simulink model "Sim_model"  (R2022b)
settings: Solver=daessc  StartTime=0.0  StopTime=10.0  RelTol=1e-5
settings Model: Creator=theko  LastModifiedBy=theko

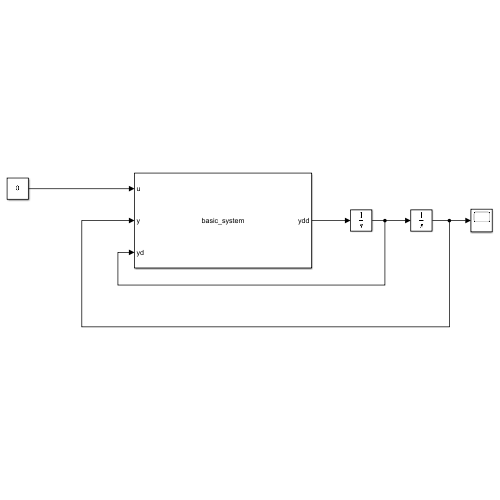
[thumbnail: Simulink's stored preview of the top-level diagram]
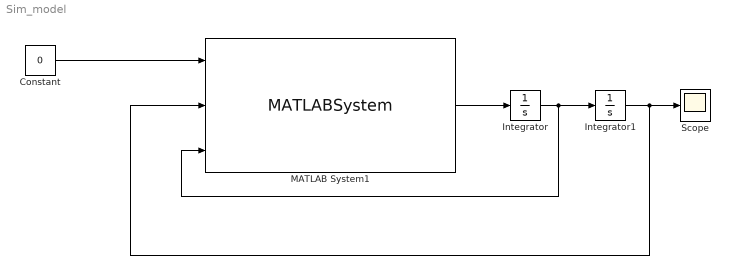
== system Sim_model ==
  Constant : Constant  Value=0
  Integrator : Integrator  InitialCondition=1
  Integrator1 : Integrator  InitialCondition=1
  MATLAB System1 : MATLABSystem  System=basic_system  m=0.5  k=10  b=1  SimulateUsing=Interpreted execution
      mask Type: basic_system
      mask Display:
      | disp('basic_system');
      | port_label('input',1,'u');
      | port_label('input',2,'y');
      | port_label('input',3,'yd');
      | port_label('output',1,'ydd');
  Scope : Scope
  wires:
  Constant/1 -> MATLAB System1/1
  Integrator/1 -> MATLAB System1/3, Integrator1/1
  MATLAB System1/1 -> Integrator/1
  Integrator1/1 -> Scope/1, MATLAB System1/2
